simulink model "torqueBalancing2012b"  (Simulink 8.0)
settings: Solver=FixedStepDiscrete  StartTime=0.0  StopTime="CONFIG.SIMULATION_TIME "  FixedStep=CONFIG.Ts  RelTol=1e-3
InitFcn:
  | cd(fileparts(which(bdroot)));
  | initTorqueBalancing;
values from neighbouring files (symbols this model uses):
  baseToWorldRotationPort = ['/' WBT_modelName '/floatingBaseRotationMatrix:i']    [initTorqueBalancing.m]
  WBT_modelName = 'matlabTorqueBalancing'    [initTorqueBalancing.m]
undefined symbols (not defined in the file or in its folder): bVectorConstraints, CONFIG, ConstraintsMatrix, DiscIntNeverNeededParam, gain, references, reg, ROBOT_DOF, ROBOT_DOF_FOR_SIMULINK, sat, SM, sm, WBT_robotName
libraries: WBToolboxLibrary x114, simulink x11
(part 1 of 3)
settings Model: Creator=daniele  LastModifiedBy=DanielePucci
settings DebuggingCC: FcnCallInpInsideContextMsg=EnableAllAsWarning  FrameProcessingCompatibilityMsg=error
settings SFSimCC: SimParseCustomCode=off
settings CodeAppCC: CustomSymbolStrType=$N$R$M_T
settings GRTTargetCC: CodeReplacementLibrary=C89/C90 (ANSI)  CombineOutputUpdateFcns=off  GRTInterface=on

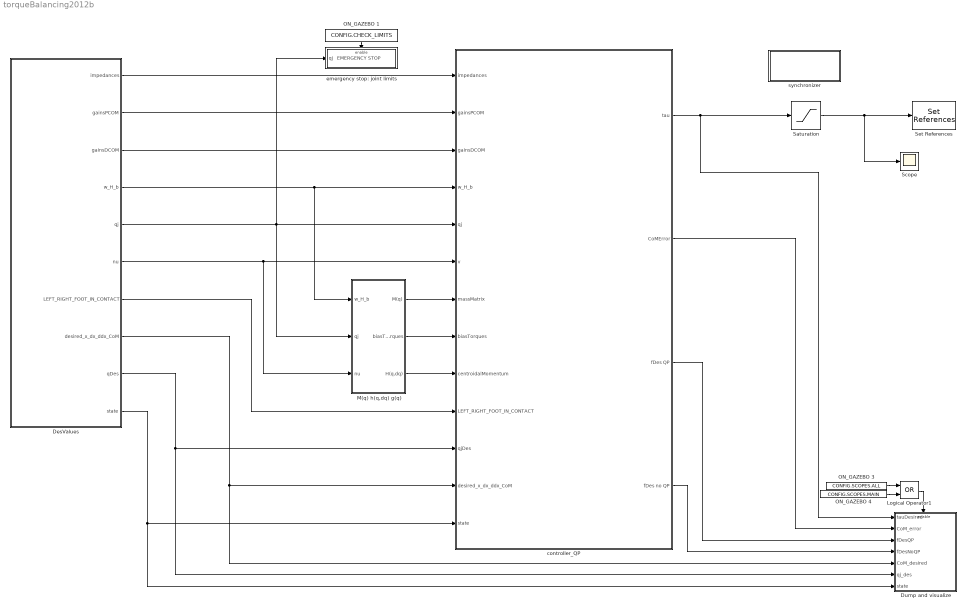
== system torqueBalancing2012b ==
  DesValues : Subsystem  Priority=-10
  Dump and visualize : Subsystem
  Logical Operator1 : Logic  Operator=OR  AllPortsSameDT=off  OutDataTypeStr=boolean
  M(q) h(q,dq) g(q) : Subsystem
  ON_GAZEBO 1 : Constant  Value=CONFIG.CHECK_LIMITS
  ON_GAZEBO 3 : Constant  Value=CONFIG.SCOPES.ALL
  ON_GAZEBO 4 : Constant  Value=CONFIG.SCOPES.MAIN
  Saturation : Saturate  UpperLimit=sat.torque  LowerLimit=-sat.torque
  Scope : Scope
      settings: TimeRange=auto  LimitDataPoints=on  MaxDataPoints=5000  SaveToWorkspace=off  YMin=-75.00000  YMax=75.00000  SampleTime=-1  DataFormat=Array
  Set References : WBToolboxLibrary/wholeBodyActuators/Set References  controlType=Torque  robotName=WBT_robotName  localName=WBT_modelName  wbiFile=WBT_wbiFilename  wbiList=WBT_wbiList
  controller_QP : Subsystem
  emergency stop: joint limits : Subsystem
  synchronizer : Subsystem
      mask Display: disp('SYNCHRONIZER')
  wires:
  M(q) h(q,dq) g(q)/1(M(q)) -> controller_QP/7(massMatrix)
  DesValues/5(qj) -> emergency stop: joint limits/1(qj   EMERGENCY STOP), controller_QP/5(qj), M(q) h(q,dq) g(q)/2(qj)
  M(q) h(q,dq) g(q)/2(biasTorques) -> controller_QP/8(biasTorques)
  M(q) h(q,dq) g(q)/3(H(q,dq)) -> controller_QP/9(centroidalMomentum)
  controller_QP/1("tau ") -> Dump and visualize/1(tauDesired), Saturation/1
  controller_QP/2(CoMError) -> Dump and visualize/2(CoM_error)
  DesValues/9(qDes) -> Dump and visualize/6(qj_des), controller_QP/11(qjDes)
  DesValues/7(LEFT_RIGHT_FOOT_IN_CONTACT) -> controller_QP/10(LEFT_RIGHT_FOOT_IN_CONTACT)
  DesValues/8(desired_x_dx_ddx_CoM) -> Dump and visualize/5(CoM_desired), controller_QP/12(desired_x_dx_ddx_CoM)
  DesValues/1(impedances) -> controller_QP/1(impedances)
  Saturation/1 -> Scope/1, Set References/1
  DesValues/4(w_H_b) -> M(q) h(q,dq) g(q)/1(w_H_b), controller_QP/4(w_H_b)
  DesValues/6(nu) -> controller_QP/6(v), M(q) h(q,dq) g(q)/3(nu)
  Logical Operator1/1 -> Dump and visualize/Enable
  DesValues/10(state) -> Dump and visualize/7(state), controller_QP/13("state ")
  controller_QP/4(fDes no QP) -> Dump and visualize/4(fDesNoQP)
  controller_QP/3(fDes QP) -> Dump and visualize/3(fDesQP)
  ON_GAZEBO 1/1 -> emergency stop: joint limits/Enable
  ON_GAZEBO 3/1 -> Logical Operator1/1
  ON_GAZEBO 4/1 -> Logical Operator1/2
  DesValues/2(gainsPCOM) -> controller_QP/2(gainsPCOM)
  DesValues/3(gainsDCOM) -> controller_QP/3(gainsDCOM)

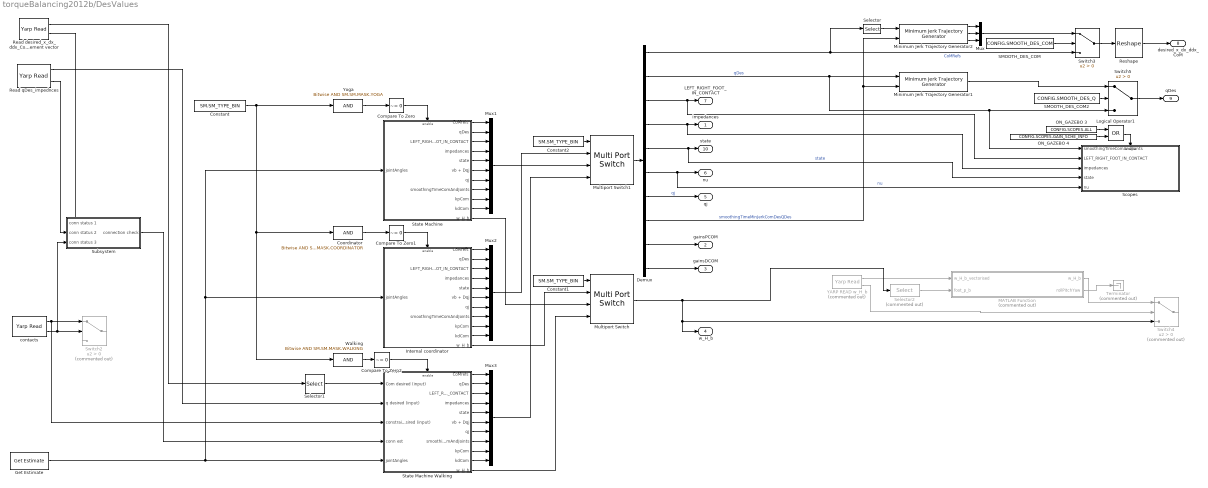
== system torqueBalancing2012b/DesValues ==
  Compare To Zero : simulink/Logic and Bit Operations/Compare To Zero  relop=~=  OutDataTypeStr=boolean
  Compare To Zero1 : simulink/Logic and Bit Operations/Compare To Zero  relop=~=  OutDataTypeStr=boolean
  Compare To Zero2 : simulink/Logic and Bit Operations/Compare To Zero  relop=~=  OutDataTypeStr=boolean
  Constant : Constant  Priority=-10  Value=SM.SM_TYPE_BIN  OutDataTypeStr=uint8
  Constant1 : Constant  Priority=-10  Value=SM.SM_TYPE_BIN  OutDataTypeStr=uint8
  Constant2 : Constant  Priority=-10  Value=SM.SM_TYPE_BIN  OutDataTypeStr=uint8
  Coordinator : simulink/Logic and Bit Operations/Bitwise Operator  logicop=AND  UseBitMask=on  BitMask=SM.SM.MASK.COORDINATOR  BitMaskRealWorld=Stored Integer
  Demux : Demux  Outputs=[9,ROBOT_DOF,2,ROBOT_DOF,1,ROBOT_DOF+6,ROBOT_DOF,1,3,3]
  Get Estimate : WBToolboxLibrary/wholeBodyStates/Get Estimate  estimateType=Joints Position  robotName=WBT_robotName  localName=WBT_modelName  wbiFile=WBT_wbiFilename  wbiList=WBT_wbiList
  Internal coordinator : Subsystem
  Logical Operator1 : Logic  Operator=OR  AllPortsSameDT=off  OutDataTypeStr=boolean
  MATLAB Function : MATLAB Function  Commented=on  TreatAsAtomicUnit=on
      settings: PermitHierarchicalResolution=ParametersOnly
  Minimum Jerk Trajectory Generator1 : WBToolboxLibrary/Utilities/Minimum Jerk Trajectory Generator  externalSettlingTime=on  settlingTime=1  sampleTime=CONFIG.Ts  firstDerivatives=off  secondDerivatives=off  explicitInitialValue=off
  Minimum Jerk Trajectory Generator2 : WBToolboxLibrary/Utilities/Minimum Jerk Trajectory Generator  externalSettlingTime=on  settlingTime=references.com.smoothingTime  sampleTime=CONFIG.Ts  firstDerivatives=on  secondDerivatives=on  explicitInitialValue=off
  Multiport Switch : MultiPortSwitch  DataPortOrder=Specify indices  DataPortIndices={1, 2, 4}
  Multiport Switch1 : MultiPortSwitch  DataPortOrder=Specify indices  DataPortIndices={1, 2, 4}
  Mux : Mux  Inputs=3
  Mux1 : Mux  Inputs=10
  Mux2 : Mux  Inputs=10
  Mux3 : Mux  Inputs=10
  ON_GAZEBO 3 : Constant  Value=CONFIG.SCOPES.ALL
  ON_GAZEBO 4 : Constant  Value=CONFIG.SCOPES.GAIN_SCHE_INFO
  Read desired_x_dx_ddx_CoM as 9 element vector : WBToolboxLibrary/Utilities/Yarp Read  portName=PORTS.COM_DES  signalSize=9  blocking=off  timestamp=off  autoconnect=off  errorOnConnection=on
  Read qDes_impednces : WBToolboxLibrary/Utilities/Yarp Read  portName=PORTS.Q_DES  signalSize=ROBOT_DOF  blocking=off  timestamp=off  autoconnect=off  errorOnConnection=on
  Reshape : Reshape  OutputDimensionality=Customize  OutputDimensions=[3,3]
  SMOOTH_DES_COM : Constant  Value=CONFIG.SMOOTH_DES_COM
  SMOOTH_DES_COM2 : Constant  Value=CONFIG.SMOOTH_DES_Q
  "Scopes  " : Subsystem
  Selector : Selector  InputPortWidth=9  IndexOptions=Index vector (dialog)  Indices=[1 2 3]  OutputSizes=1
  Selector1 : Selector  InputPortWidth=9  IndexOptions=Index vector (dialog)  Indices=[1 2 3]  OutputSizes=1
  Selector2 : Selector  Commented=on  NumberOfDimensions=2  InputPortWidth=3  IndexOptions=Index vector (dialog),Index vector (dialog)  Indices=[1 2 3],4  OutputSizes=1,1
  State Machine : Subsystem  Priority=-100
  State Machine Walking : Subsystem  Priority=-100
  Subsystem : Subsystem
  Switch2 : Switch  Commented=on  Criteria=u2 > Threshold
  Switch3 : Switch  Criteria=u2 > Threshold
  Switch4 : Switch  Commented=on  Criteria=u2 > Threshold
  Switch5 : Switch  Criteria=u2 > Threshold
  Terminator : Terminator  Commented=on
  Walking : simulink/Logic and Bit Operations/Bitwise Operator  logicop=AND  UseBitMask=on  BitMask=SM.SM.MASK.WALKING  BitMaskRealWorld=Stored Integer
  YARP READ w_H_b : WBToolboxLibrary/Utilities/Yarp Read  Commented=on  portName=[baseToWorldRotationPort]  signalSize=16  blocking=off  timestamp=off  autoconnect=off  errorOnConnection=on
  Yoga : simulink/Logic and Bit Operations/Bitwise Operator  logicop=AND  UseBitMask=on  BitMask=SM.SM.MASK.YOGA  BitMaskRealWorld=Stored Integer
  contacts : WBToolboxLibrary/Utilities/Yarp Read  portName=['/' WBT_modelName '/constraints:i']  signalSize=2  blocking=off  timestamp=off  autoconnect=off  errorOnConnection=on
  impedances : Outport
  gainsPCOM : Outport  Port=2
  gainsDCOM : Outport  Port=3
  w_H_b : Outport  Port=4
  qj : Outport  Port=5
  nu : Outport  Port=6
  LEFT_RIGHT_FOOT_IN_CONTACT : Outport  Port=7
  desired_x_dx_ddx_CoM : Outport  Port=8
  qDes : Outport  Port=9
  state : Outport  Port=10
  wires:
  Read desired_x_dx_ddx_CoM as 9 element vector/2 -> Subsystem/1(conn status 1)
  Read desired_x_dx_ddx_CoM as 9 element vector/1 -> Selector1/1
  Reshape/1 -> desired_x_dx_ddx_CoM/1
  Read qDes_impednces/2 -> Subsystem/2(conn status 2)
  contacts/2 -> Subsystem/3(conn status 3), Switch2/2
  Minimum Jerk Trajectory Generator2/1 -> Mux/1
  Minimum Jerk Trajectory Generator2/2 -> Mux/2
  Minimum Jerk Trajectory Generator2/3 -> Mux/3
  Switch3/1 -> Reshape/1
  SMOOTH_DES_COM/1 -> Switch3/2
  SMOOTH_DES_COM2/1 -> Switch5/2
  Switch5/1 -> qDes/1
  Constant/1 -> Walking/1, Coordinator/1, Yoga/1
  State Machine/3(LEFT_RIGHT_FOOT_IN_CONTACT) -> Mux1/3
  State Machine/2(qDes) -> Mux1/2
  State Machine/1(CoMrefs) -> Mux1/1
  Internal coordinator/1(CoMrefs) -> Mux2/1
  Internal coordinator/2(qDes) -> Mux2/2
  Internal coordinator/3(LEFT_RIGHT_FOOT_IN_CONTACT) -> Mux2/3
  State Machine/4(impedances) -> Mux1/4
  Internal coordinator/4(impedances) -> Mux2/4
  State Machine/5(state) -> Mux1/5
  Internal coordinator/5(state) -> Mux2/5
  Internal coordinator/6(vb + Dqj) -> Mux2/6
  Internal coordinator/7(qj) -> Mux2/7
  State Machine/6(vb + Dqj) -> Mux1/6
  State Machine/7(qj) -> Mux1/7
  Demux/7 -> qj/1  "qj"
  State Machine Walking/4(impedances) -> Mux3/4
  State Machine Walking/3(LEFT_RIGHT_FOOT_IN_CONTACT) -> Mux3/3
  State Machine Walking/5(state) -> Mux3/5
  State Machine Walking/6(vb + Dqj) -> Mux3/6
  State Machine Walking/1(CoMrefs) -> Mux3/1
  State Machine Walking/7(qj) -> Mux3/7
  Coordinator/1 -> Compare To Zero1/1
  Yoga/1 -> Compare To Zero/1
  Walking/1 -> Compare To Zero2/1
  Mux3/1 -> Multiport Switch1/4
  State Machine Walking/11(w_H_b) -> Multiport Switch/4
  Selector1/1 -> State Machine Walking/1(Com desired (input))
  Compare To Zero/1 -> State Machine/Enable
  Compare To Zero1/1 -> Internal coordinator/Enable
  Compare To Zero2/1 -> State Machine Walking/Enable
  Mux1/1 -> Multiport Switch1/3
  Mux2/1 -> Multiport Switch1/2
  State Machine/11(w_H_b) -> Multiport Switch/3
  Internal coordinator/11(w_H_b) -> Multiport Switch/2
  Read qDes_impednces/1 -> State Machine Walking/2(q desired (input))
  Subsystem/1(connection check) -> State Machine Walking/4(conn est)
  State Machine Walking/2(qDes) -> Mux3/2
  contacts/1 -> State Machine Walking/3(constraints desired (input)), Switch2/1
  YARP READ w_H_b/1 -> MATLAB Function/1(w_H_b_vectorised)
  MATLAB Function/1(w_H_b) -> Switch4/1
  Selector2/1 -> MATLAB Function/2(foot_p_b)
  Multiport Switch/1 -> Selector2/1, Switch4/3, w_H_b/1
  YARP READ w_H_b/2 -> Switch4/2
  MATLAB Function/2(rollPitchYaw) -> Terminator/1
  Demux/5 -> "Scopes  "/4(state), state/1  "state"
  Internal coordinator/8(smoothingTimeComAndJoints) -> Mux2/8
  State Machine Walking/8(smoothingTimeComAndJoints) -> Mux3/8
  State Machine/8(smoothingTimeComAndJoints) -> Mux1/8
  Demux/8 -> Minimum Jerk Trajectory Generator2/2, Minimum Jerk Trajectory Generator1/2  "smoothingTimeMinJerkComDesQDes"
  Logical Operator1/1 -> "Scopes  "/Enable
  Demux/1 -> Selector/1, Switch3/3  "CoMRefs"
  Mux/1 -> Switch3/1
  Selector/1 -> Minimum Jerk Trajectory Generator2/1
  Demux/2 -> Minimum Jerk Trajectory Generator1/1, "Scopes  "/1(smoothingTimeComAndJoints), Switch5/3  "qDes"
  Minimum Jerk Trajectory Generator1/1 -> Switch5/1
  ON_GAZEBO 3/1 -> Logical Operator1/1
  ON_GAZEBO 4/1 -> Logical Operator1/2
  Demux/6 -> nu/1, "Scopes  "/5(nu)  "nu"
  Get Estimate/1 -> State Machine/1(jointAngles), Internal coordinator/1(jointAngles), State Machine Walking/5(jointAngles)
  State Machine/9(kpCom) -> Mux1/9
  State Machine/10(kdCom) -> Mux1/10
  Internal coordinator/9(kpCom) -> Mux2/9
  Internal coordinator/10(kdCom) -> Mux2/10
  State Machine Walking/9(kpCom) -> Mux3/9
  State Machine Walking/10(kdCom) -> Mux3/10
  Multiport Switch1/1 -> Demux/1
  Demux/4 -> "Scopes  "/3(impedances), impedances/1
  Demux/3 -> "Scopes  "/2(LEFT_RIGHT_FOOT_IN_CONTACT), LEFT_RIGHT_FOOT_IN_CONTACT/1
  Demux/9 -> gainsPCOM/1
  Demux/10 -> gainsDCOM/1
  Constant1/1 -> Multiport Switch/1
  Constant2/1 -> Multiport Switch1/1

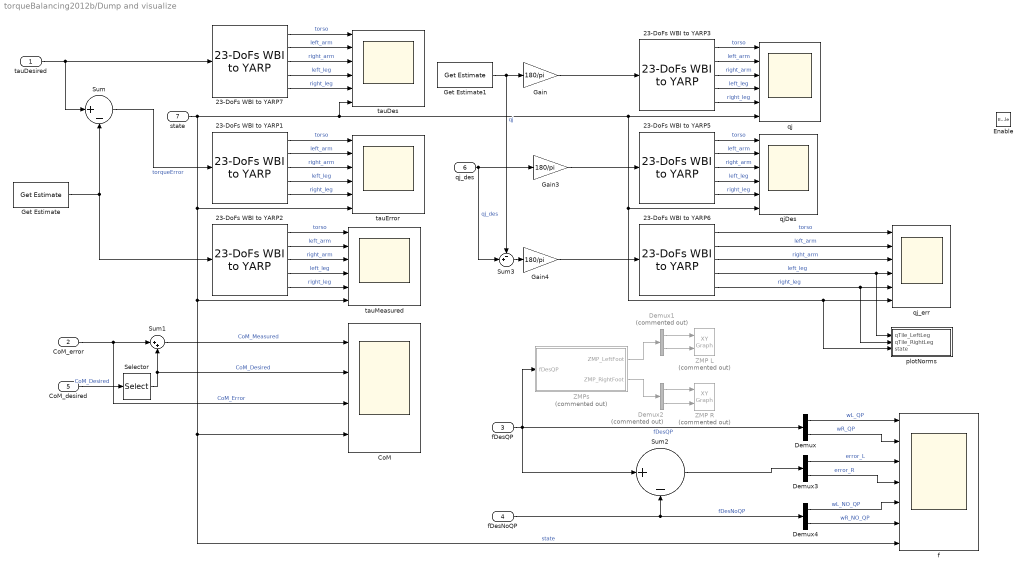
== system torqueBalancing2012b/Dump and visualize ==
  tauDesired : Inport
  CoM_error : Inport  Port=2
  fDesQP : Inport  Port=3
  fDesNoQP : Inport  Port=4
  CoM_desired : Inport  Port=5
  qj_des : Inport  Port=6
  state : Inport  Port=7
  Enable : EnablePort
  23-DoFs WBI to YARP{1..3,5..7} (6 alike) : WBToolboxLibrary/Utilities/23-DoFs WBI to YARP
  CoM : Scope  NumInputPorts=4
      settings: TimeRange=400  ShowLegends=on  MaxDataPoints=5000  SaveToWorkspace=off  SaveName=CoM_data  YMin=-0.89345~-0.34739~-1.03525~0.625  YMax=1.44665~1.31967~1.03732~4.375  SampleTime=-1
  Demux : Demux  Outputs=2
  Demux1 : Demux  Commented=on  Outputs=2
  Demux2 : Demux  Commented=on  Outputs=2
  Demux3 : Demux  Outputs=2
  Demux4 : Demux  Outputs=2
  Gain : Gain  Gain=180/pi
  Gain3 : Gain  Gain=180/pi
  Gain4 : Gain  Gain=180/pi
  Get Estimate : WBToolboxLibrary/wholeBodyStates/Get Estimate  estimateType=Joints Torque  robotName=WBT_robotName  localName=WBT_modelName  wbiFile=WBT_wbiFilename  wbiList=WBT_wbiList
  Get Estimate1 : WBToolboxLibrary/wholeBodyStates/Get Estimate  estimateType=Joints Position  robotName=WBT_robotName  localName=WBT_modelName  wbiFile=WBT_wbiFilename  wbiList=WBT_wbiList
  Selector : Selector  NumberOfDimensions=2  IndexOptions=Index vector (dialog),Index vector (dialog)  Indices=[1:3],1  OutputSizes=1,1
  Sum : Sum  Inputs=|+-
  Sum1 : Sum  Inputs=|++
  Sum2 : Sum  Inputs=|+-
  Sum3 : Sum  Inputs=-+|
  ZMP L : simulink/Sinks/XY Graph  Commented=on  xmin=gain.footSize(1,1)  xmax=gain.footSize(1,2)  ymin=gain.footSize(2,1)  ymax=gain.footSize(2,2)  st=-1
  ZMP R : simulink/Sinks/XY Graph  Commented=on  xmin=gain.footSize(1,1)  xmax=gain.footSize(1,2)  ymin=gain.footSize(2,1)  ymax=gain.footSize(2,2)  st=-1
  ZMPs : Subsystem  Commented=on
  f : Scope  NumInputPorts=7
      settings: TimeRange=40  MaxDataPoints=5000  SaveToWorkspace=off  SaveName=ScopeData2  YMin=-58.62138~-58.62138~-58.62138~-58.62138~-58.62138~-58.62138~-58.62138  YMax=275.46472~275.46472~275.46472~275.46472~275.46472~275.46472~275.46472  SampleTime=-1  DataFormat=Array
  plotNorms : Subsystem
  qj : Scope  NumInputPorts=6
      settings: TimeRange=40  ShowLegends=on  MaxDataPoints=5000  SaveToWorkspace=off  SaveName=qj_and_v  YMin=-27.84492~-27.84492~-27.84492~-27.84492~-27.84492~-27.84492  YMax=29.50386~29.50386~29.50386~29.50386~29.50386~29.50386  SampleTime=-1
  qjDes : Scope  NumInputPorts=6
      settings: TimeRange=40  ShowLegends=on  MaxDataPoints=5000  SaveToWorkspace=off  SaveName=qj_and_v3  YMin=-30.77436~-30.77436~-30.77436~-30.77436~-30.77436~-30.77436  YMax=32.14439~32.14439~32.14439~32.14439~32.14439~32.14439  SampleTime=-1
  qj_err : Scope  NumInputPorts=6
      settings: TimeRange=40  ShowLegends=on  MaxDataPoints=5000  SaveToWorkspace=off  SaveName=qj_and_v4  YMin=-19.07921~-19.07921~-19.07921~-19.07921~-19.07921~-19.07921  YMax=25.04716~25.04716~25.04716~25.04716~25.04716~25.04716  SampleTime=-1
  tauDes : Scope  NumInputPorts=6
      settings: TimeRange=14  ShowLegends=on  MaxDataPoints=5000  SaveToWorkspace=off  SaveName=tauDes  YMin=-11.78546~-11.78546~-11.78546~-11.78546~-11.78546~-11.78546  YMax=8.52242~8.52242~8.52242~8.52242~8.52242~8.52242  SampleTime=-1
  tauError : Scope  NumInputPorts=6
      settings: TimeRange=90  ShowLegends=on  MaxDataPoints=5000  SaveToWorkspace=off  SaveName=tauError  YMin=-9.6915~-5.81436~-6.54838~-48.80934~-49.21526~-0.5  YMax=9.49753~5.53968~7.62852~37.43254~39.21906~14.5  SampleTime=-1
  tauMeasured : Scope  NumInputPorts=6
      settings: TimeRange=14  ShowLegends=on  MaxDataPoints=5000  SaveToWorkspace=off  SaveName=tauMeasured  YMin=-10.14812~-10.14812~-10.14812~-10.14812~-10.14812~-10.14812  YMax=9.97513~9.97513~9.97513~9.97513~9.97513~9.97513  SampleTime=-1
  wires:
  CoM_error/1 -> Sum1/1, CoM/3  "CoM_Error"
  CoM_desired/1 -> Selector/1  "CoM_Desired"
  Sum1/1 -> CoM/1  "CoM_Measured"
  Get Estimate1/1 -> Sum3/1, Gain/1  "qj"
  Gain/1 -> 23-DoFs WBI to YARP3/1
  23-DoFs WBI to YARP3/5 -> qj/5  "right_leg"
  23-DoFs WBI to YARP3/1 -> qj/1  "torso"
  23-DoFs WBI to YARP3/2 -> qj/2  "left_arm"
  23-DoFs WBI to YARP3/4 -> qj/4  "left_leg"
  23-DoFs WBI to YARP3/3 -> qj/3  "right_arm"
  fDesQP/1 -> Demux/1, ZMPs/1(fDesQP), Sum2/1  "fDesQP"
  ZMPs/1(ZMP_LeftFoot) -> Demux1/1
  ZMPs/2(ZMP_RightFoot) -> Demux2/1
  Demux1/1 -> ZMP L/1
  Demux1/2 -> ZMP L/2
  Demux2/1 -> ZMP R/1
  Demux2/2 -> ZMP R/2
  Sum2/1 -> Demux3/1
  fDesNoQP/1 -> Demux4/1, Sum2/2  "fDesNoQP"
  tauDesired/1 -> 23-DoFs WBI to YARP7/1, Sum/1
  Get Estimate/1 -> 23-DoFs WBI to YARP2/1, Sum/2
  23-DoFs WBI to YARP7/5 -> tauDes/5  "right_leg"
  23-DoFs WBI to YARP7/1 -> tauDes/1  "torso"
  23-DoFs WBI to YARP7/2 -> tauDes/2  "left_arm"
  23-DoFs WBI to YARP7/4 -> tauDes/4  "left_leg"
  23-DoFs WBI to YARP7/3 -> tauDes/3  "right_arm"
  23-DoFs WBI to YARP1/5 -> tauError/5  "right_leg"
  23-DoFs WBI to YARP1/1 -> tauError/1  "torso"
  23-DoFs WBI to YARP1/2 -> tauError/2  "left_arm"
  23-DoFs WBI to YARP1/4 -> tauError/4  "left_leg"
  23-DoFs WBI to YARP1/3 -> tauError/3  "right_arm"
  Sum/1 -> 23-DoFs WBI to YARP1/1  "torqueError"
  23-DoFs WBI to YARP2/5 -> tauMeasured/5  "right_leg"
  23-DoFs WBI to YARP2/1 -> tauMeasured/1  "torso"
  23-DoFs WBI to YARP2/2 -> tauMeasured/2  "left_arm"
  23-DoFs WBI to YARP2/4 -> tauMeasured/4  "left_leg"
  23-DoFs WBI to YARP2/3 -> tauMeasured/3  "right_arm"
  qj_des/1 -> Sum3/2, Gain3/1  "qj_des"
  Gain3/1 -> 23-DoFs WBI to YARP5/1
  23-DoFs WBI to YARP5/5 -> qjDes/5  "right_leg"
  23-DoFs WBI to YARP5/1 -> qjDes/1  "torso"
  23-DoFs WBI to YARP5/2 -> qjDes/2  "left_arm"
  23-DoFs WBI to YARP5/4 -> qjDes/4  "left_leg"
  23-DoFs WBI to YARP5/3 -> qjDes/3  "right_arm"
  Gain4/1 -> 23-DoFs WBI to YARP6/1
  23-DoFs WBI to YARP6/5 -> plotNorms/2(qTile_RightLeg), qj_err/5  "right_leg"
  23-DoFs WBI to YARP6/1 -> qj_err/1  "torso"
  23-DoFs WBI to YARP6/2 -> qj_err/2  "left_arm"
  23-DoFs WBI to YARP6/4 -> plotNorms/1(qTile_LeftLeg), qj_err/4  "left_leg"
  23-DoFs WBI to YARP6/3 -> qj_err/3  "right_arm"
  Sum3/1 -> Gain4/1
  Selector/1 -> Sum1/2, CoM/2  "CoM_Desired"
  state/1 -> tauDes/6, plotNorms/3(state), qj_err/6, qjDes/6, qj/6, f/7, CoM/4, tauMeasured/6, tauError/6  "state"
  Demux/1 -> f/1  "wL_QP"
  Demux/2 -> f/2  "wR_QP"
  Demux3/1 -> f/3  "error_L"
  Demux3/2 -> f/4  "error_R"
  Demux4/1 -> f/5  "wL_NO_QP"
  Demux4/2 -> f/6  "wR_NO_QP"

== system torqueBalancing2012b/M(q) h(q,dq) g(q) ==
  w_H_b : Inport
  qj : Inport  Port=2
  nu : Inport  Port=3
  Centroidal Momentum : WBToolboxLibrary/wholeBodyModel/Dynamics/Centroidal Momentum  robotName=WBT_robotName  localName=WBT_modelName  wbiFile=WBT_wbiFilename  wbiList=WBT_wbiList
  "CoM6D ->  CoMXYZ1" : Selector  InputPortWidth=6+ROBOT_DOF  IndexOptions=Index vector (dialog)  Indices=[7:6+ROBOT_DOF]  OutputSizes=1
  "CoM6D ->  CoMXYZ2" : Selector  InputPortWidth=6+ROBOT_DOF  IndexOptions=Index vector (dialog)  Indices=[1 2 3 4 5 6]  OutputSizes=1
  Get Bias Forces : WBToolboxLibrary/wholeBodyModel/Dynamics/Get Bias Forces  robotName=WBT_robotName  localName=WBT_modelName  wbiFile=WBT_wbiFilename  wbiList=WBT_wbiList  explicitGravity=off
  Mass Matrix : WBToolboxLibrary/wholeBodyModel/Dynamics/Mass Matrix  robotName=WBT_robotName  localName=WBT_modelName  wbiFile=WBT_wbiFilename  wbiList=WBT_wbiList
  M(q) : Outport
  biasTorques : Outport  Port=2
  H(q,dq) : Outport  Port=3
  wires:
  Mass Matrix/1 -> M(q)/1
  Centroidal Momentum/1 -> H(q,dq)/1
  Get Bias Forces/1 -> biasTorques/1
  w_H_b/1 -> Centroidal Momentum/1, Get Bias Forces/1, Mass Matrix/1
  qj/1 -> Centroidal Momentum/2, Get Bias Forces/2, Mass Matrix/2
  "CoM6D ->  CoMXYZ2"/1 -> Centroidal Momentum/3, Get Bias Forces/3
  "CoM6D ->  CoMXYZ1"/1 -> Get Bias Forces/4, Centroidal Momentum/4
  nu/1 -> "CoM6D ->  CoMXYZ1"/1, "CoM6D ->  CoMXYZ2"/1

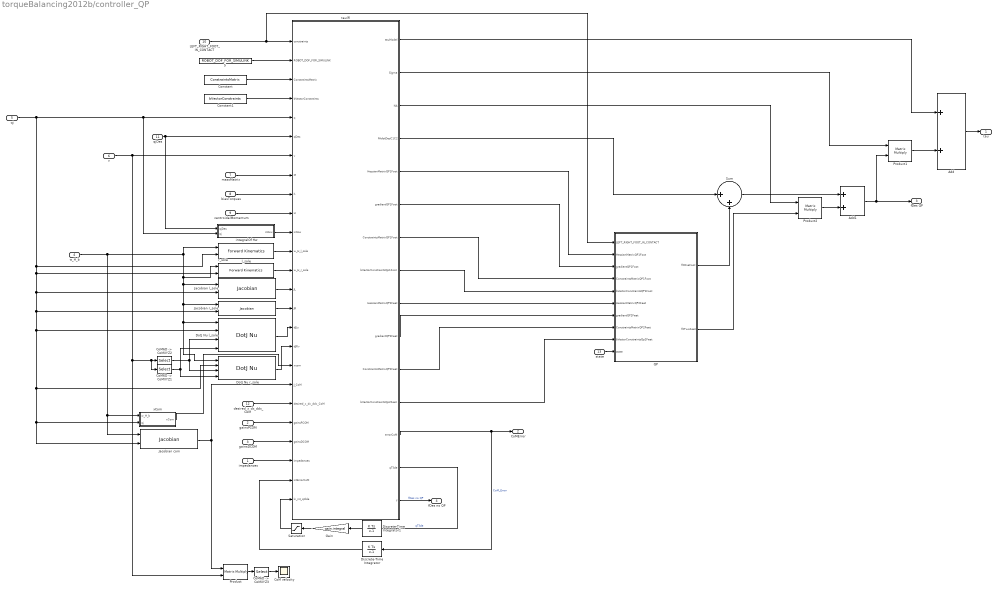
== system torqueBalancing2012b/controller_QP ==
  impedances : Inport
  gainsPCOM : Inport  Port=2
  gainsDCOM : Inport  Port=3
  w_H_b : Inport  Port=4
  qj : Inport  Port=5
  v : Inport  Port=6
  massMatrix : Inport  Port=7
  biasTorques : Inport  Port=8
  centroidalMomentum : Inport  Port=9
  LEFT_RIGHT_FOOT_IN_CONTACT : Inport  Port=10
  qjDes : Inport  Port=11
  desired_x_dx_ddx_CoM : Inport  Port=12
  "state " : Inport  Port=13
  "    5" : Constant  Value=ROBOT_DOF_FOR_SIMULINK
  Add : Sum
  Add1 : Sum
  CoM velocity : Scope
      settings: TimeRange=auto  MaxDataPoints=5000  SaveToWorkspace=off  SaveName=ScopeData3  YMin=-0.13469  YMax=0.38733  SampleTime=-1
  "CoM6D ->  CoMXYZ1" : Selector  InputPortWidth=6+ROBOT_DOF  IndexOptions=Index vector (dialog)  Indices=[7:6+ROBOT_DOF]  OutputSizes=1
  "CoM6D ->  CoMXYZ2" : Selector  InputPortWidth=6+ROBOT_DOF  IndexOptions=Index vector (dialog)  Indices=[1 2 3 4 5 6]  OutputSizes=1
  "CoM6D ->  CoMXYZ3" : Selector  InputPortWidth=6  IndexOptions=Index vector (dialog)  Indices=[1 2 3]  OutputSizes=1
  Constant : Constant  Value=ConstraintsMatrix
  Constant1 : Constant  Value=bVectorConstraints
  Discrete-Time Integrator : DiscreteIntegrator  InitialCondition=[0 0 0]  SampleTime=CONFIG.Ts  ICPrevOutput=DiscIntNeverNeededParam  ICPrevScaledInput=DiscIntNeverNeededParam
  Discrete-Time Integrator1 : DiscreteIntegrator  InitialCondition=zeros(ROBOT_DOF,1)  SampleTime=CONFIG.Ts  ICPrevOutput=DiscIntNeverNeededParam  ICPrevScaledInput=DiscIntNeverNeededParam
  "DotJ Nu l_sole " : WBToolboxLibrary/wholeBodyModel/Jacobians/DotJ Nu  frameName='l_sole'  robotName=WBT_robotName  localName=WBT_modelName  wbiFile=WBT_wbiFilename  wbiList=WBT_wbiList
  "DotJ Nu r_sole " : WBToolboxLibrary/wholeBodyModel/Jacobians/DotJ Nu  frameName='r_sole'  robotName=WBT_robotName  localName=WBT_modelName  wbiFile=WBT_wbiFilename  wbiList=WBT_wbiList
  Gain : Gain  Gain=gain.integral
  Jacobian com : WBToolboxLibrary/wholeBodyModel/Jacobians/Jacobian  frameName='com'  robotName=WBT_robotName  localName=WBT_modelName  wbiFile=WBT_wbiFilename  wbiList=WBT_wbiList
  Jacobian l_sole : WBToolboxLibrary/wholeBodyModel/Jacobians/Jacobian  frameName='l_sole'  robotName=WBT_robotName  localName=WBT_modelName  wbiFile=WBT_wbiFilename  wbiList=WBT_wbiList
  Jacobian r_sole : WBToolboxLibrary/wholeBodyModel/Jacobians/Jacobian  frameName='r_sole'  robotName=WBT_robotName  localName=WBT_modelName  wbiFile=WBT_wbiFilename  wbiList=WBT_wbiList
  Product : Product  Multiplication=Matrix(*)
  Product1 : Product  Multiplication=Matrix(*)
  Product2 : Product  Multiplication=Matrix(*)
  QP : Subsystem
  Saturation : Saturate  UpperLimit=sat.integral  LowerLimit=-sat.integral
  Sum : Sum  Inputs=|++
  integralOf Hw : Subsystem
  l_sole : WBToolboxLibrary/wholeBodyModel/Kinematics/Forward Kinematics  frameName='l_sole'  robotName=WBT_robotName  localName=WBT_modelName  wbiFile=WBT_wbiFilename  wbiList=WBT_wbiList
  r_sole : WBToolboxLibrary/wholeBodyModel/Kinematics/Forward Kinematics  frameName='r_sole'  robotName=WBT_robotName  localName=WBT_modelName  wbiFile=WBT_wbiFilename  wbiList=WBT_wbiList
  "tau(f) " : MATLAB Function  TreatAsAtomicUnit=on
      settings: PermitHierarchicalResolution=ParametersOnly
  xCom : Subsystem
  "tau " : Outport
  CoMError : Outport  Port=2
  fDes QP : Outport  Port=3
  fDes no QP : Outport  Port=4
  wires:
  LEFT_RIGHT_FOOT_IN_CONTACT/1 -> QP/1(LEFT_RIGHT_FOOT_IN_CONTACT), "tau(f) "/1(constraints)
  Discrete-Time Integrator/1 -> "tau(f) "/24(intErrorCoM)
  "tau(f) "/13(errorCoM) -> CoMError/1, Discrete-Time Integrator/1  "CoM_Error"
  Discrete-Time Integrator1/1 -> Gain/1
  "tau(f) "/14(qTilde) -> Discrete-Time Integrator1/1  "qTilde"
  Gain/1 -> Saturation/1
  Saturation/1 -> "tau(f) "/25(ki_int_qtilde)
  qj/1 -> l_sole/2, xCom/2(qj), Jacobian com/2, "DotJ Nu r_sole "/2, "DotJ Nu l_sole "/2, Jacobian r_sole/2, Jacobian l_sole/2, r_sole/2, integralOf Hw/2(qj), "tau(f) "/5(q)
  qjDes/1 -> integralOf Hw/1(qjDes), "tau(f) "/6(qDes)
  massMatrix/1 -> "tau(f) "/8(M)
  biasTorques/1 -> "tau(f) "/9(h)
  desired_x_dx_ddx_CoM/1 -> "tau(f) "/20(desired_x_dx_ddx_CoM)
  impedances/1 -> "tau(f) "/23(impedances)
  centroidalMomentum/1 -> "tau(f) "/10(H)
  r_sole/1 -> "tau(f) "/13(w_H_r_sole)
  l_sole/1 -> "tau(f) "/12(w_H_l_sole)
  Jacobian l_sole/1 -> "tau(f) "/14(JL)
  Jacobian r_sole/1 -> "tau(f) "/15(JR)
  Jacobian com/1 -> Product/1, "tau(f) "/19(J_CoM)
  "tau(f) "/5(HessianMatrixQP1Foot) -> QP/2(HessianMatrixQP1Foot)
  "tau(f) "/6(gradientQP1Foot) -> QP/3(gradientQP1Foot)
  "tau(f) "/9(HessianMatrixQP2Feet) -> QP/6(HessianMatrixQP2Feet)
  "tau(f) "/10(gradientQP2Feet) -> QP/7(gradientQP2Feet)
  "tau(f) "/11(ConstraintsMatrixQP2Feet) -> QP/8(ConstraintsMatrixQP2Feet)
  "tau(f) "/12(bVectorConstraintsQp2Feet) -> QP/9(bVectorConstraintsQp2Feet)
  "tau(f) "/4(fHdotDesC1C2) -> Sum/1
  QP/1(f0OneFoot) -> Sum/2
  Product1/1 -> Add/2
  "tau(f) "/1(tauModel) -> Add/1
  Add/1 -> "tau "/1
  Add1/1 -> fDes QP/1, Product1/2
  "    5"/1 -> "tau(f) "/2(ROBOT_DOF_FOR_SIMULINK)
  Constant/1 -> "tau(f) "/3(ConstraintsMatrix)
  Constant1/1 -> "tau(f) "/4(bVectorConstraints)
  "tau(f) "/7(ConstraintsMatrixQP1Foot) -> QP/4(ConstraintsMatrixQP1Foot)
  "tau(f) "/8(bVectorConstraintsQp1Foot) -> QP/5(bVectorConstraintsQP1Foot)
  Sum/1 -> Add1/1
  Product2/1 -> Add1/2
  "tau(f) "/3(NA) -> Product2/1
  "tau(f) "/2(Sigma) -> Product1/1
  "tau(f) "/15(f) -> fDes no QP/1  "fDes no QP"
  "DotJ Nu l_sole "/1 -> "tau(f) "/16(dJLv)
  "DotJ Nu r_sole "/1 -> "tau(f) "/17(dJRv)
  xCom/1(xCom) -> "tau(f) "/18(xcom)
  "CoM6D ->  CoMXYZ2"/1 -> "DotJ Nu r_sole "/3, "DotJ Nu l_sole "/3
  "CoM6D ->  CoMXYZ1"/1 -> "DotJ Nu r_sole "/4, "DotJ Nu l_sole "/4
  w_H_b/1 -> xCom/1(w_H_b), Jacobian com/1, r_sole/1, "DotJ Nu r_sole "/1, "DotJ Nu l_sole "/1, Jacobian r_sole/1, Jacobian l_sole/1, l_sole/1
  QP/2(f0TwoFeet) -> Product2/2
  integralOf Hw/1(intHw) -> "tau(f) "/11(intHw)
  "state "/1 -> QP/10(state)
  v/1 -> Product/2, "CoM6D ->  CoMXYZ1"/1, "CoM6D ->  CoMXYZ2"/1, "tau(f) "/7(v)
  Product/1 -> "CoM6D ->  CoMXYZ3"/1
  "CoM6D ->  CoMXYZ3"/1 -> CoM velocity/1
  gainsPCOM/1 -> "tau(f) "/21(gainsPCOM)
  gainsDCOM/1 -> "tau(f) "/22(gainsDCOM)

== system torqueBalancing2012b/emergency stop: joint limits ==
  qj   EMERGENCY STOP : Inport
  Enable : EnablePort
  Assertion : Assertion
  Get Limits : WBToolboxLibrary/wholeBodyStates/Get Limits  limitsType=Position  robotName=WBT_robotName  localName=WBT_modelName  wbiFile=WBT_wbiFilename  wbiList=WBT_wbiList
  MATLAB Function : MATLAB Function  TreatAsAtomicUnit=on
      settings: PermitHierarchicalResolution=ParametersOnly
  index1 : Constant  Value=0.01  VectorParams1D=off
  wires:
  Get Limits/1 -> MATLAB Function/1(umin)
  Get Limits/2 -> MATLAB Function/2(umax)
  index1/1 -> MATLAB Function/4(tol)
  qj   EMERGENCY STOP/1 -> MATLAB Function/3(u)
  MATLAB Function/1(inRange) -> Assertion/1

== system torqueBalancing2012b/synchronizer ==
  GAZEBO_SYNCHRONIZER : Subsystem
  Logical Operator : Logic  Operator=NOT  AllPortsSameDT=off  OutDataTypeStr=boolean
  "ON_GAZEBO " : Constant  Value=CONFIG.ON_GAZEBO
  REAL_TIME_SYNC : Subsystem
  wires:
  Logical Operator/1 -> REAL_TIME_SYNC/Enable
  "ON_GAZEBO "/1 -> GAZEBO_SYNCHRONIZER/Enable, Logical Operator/1

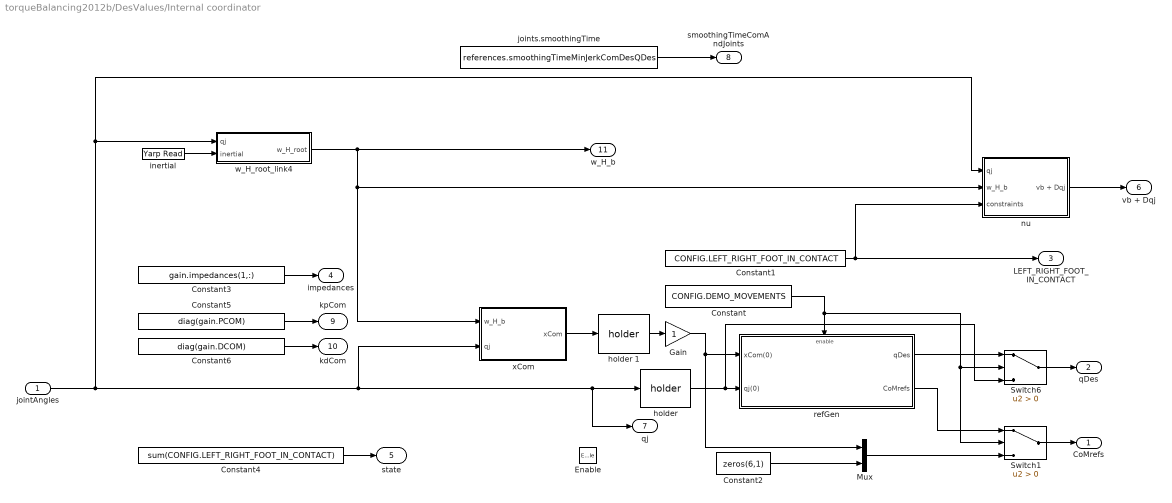
== system torqueBalancing2012b/DesValues/Internal coordinator ==
  jointAngles : Inport
  Enable : EnablePort
  Constant : Constant  Value=CONFIG.DEMO_MOVEMENTS
  Constant1 : Constant  Value=CONFIG.LEFT_RIGHT_FOOT_IN_CONTACT
  Constant2 : Constant  Value=zeros(6,1)
  Constant3 : Constant  Value=gain.impedances(1,:)
  Constant4 : Constant  Value=sum(CONFIG.LEFT_RIGHT_FOOT_IN_CONTACT)
  Constant5 : Constant  Value=diag(gain.PCOM)
  Constant6 : Constant  Value=diag(gain.DCOM)
  Gain : Gain
  Mux : Mux  Inputs=2
  Switch1 : Switch  Criteria=u2 > Threshold
  Switch6 : Switch  Criteria=u2 > Threshold
  "holder " : WBToolboxLibrary/Utilities/holder 
  holder 1 : WBToolboxLibrary/Utilities/holder 
  inertial : WBToolboxLibrary/Utilities/Yarp Read  portName=PORTS.IMU  signalSize=12  blocking=off  timestamp=off  autoconnect=on  errorOnConnection=on
  joints.smoothingTime : Constant  Value=references.smoothingTimeMinJerkComDesQDes
  nu : Subsystem
  refGen : Subsystem
  w_H_root_link4 : Subsystem  mask{link_name='l_sole'}
      mask prompts: link_name "link name"
      mask help:
      | This block evaluates the homogeneous transformation between the world and the root link, i.e. ^wH_b. It assumes that the link specified by the variable 'link_name' has a constant position
      | w.r.t. an inertial frame, but it can rotate arbitrarily. This rotation is retrived from the IMU sensor.
      mask Display:
      | str = strrep(link_name, '_','\_');
      | port_label('output',1,['{}^{',str '}H_{root}'],'texmode','on')
      | clear str;
      | 
      | port_label('input',1,'q_j','texmode','on')
      | 
      | port_label('input',2,'inertial','texmode','on')
  xCom : Subsystem
  CoMrefs : Outport
  qDes : Outport  Port=2
  LEFT_RIGHT_FOOT_IN_CONTACT : Outport  Port=3
  impedances : Outport  Port=4
  state : Outport  Port=5
  vb + Dqj : Outport  Port=6
  qj : Outport  Port=7
  smoothingTimeComAndJoints : Outport  Port=8
  kpCom : Outport  Port=9
  kdCom : Outport  Port=10
  w_H_b : Outport  Port=11
  wires:
  Constant1/1 -> nu/3("constraints "), LEFT_RIGHT_FOOT_IN_CONTACT/1
  "holder "/1 -> Switch6/3, refGen/2(qj(0))
  Constant/1 -> Switch1/2, Switch6/2, refGen/Enable
  Switch6/1 -> qDes/1
  Switch1/1 -> CoMrefs/1
  refGen/1(qDes) -> Switch6/1
  refGen/2(CoMrefs) -> Switch1/1
  Mux/1 -> Switch1/3
  Constant2/1 -> Mux/2
  Constant3/1 -> impedances/1
  Constant4/1 -> state/1
  nu/1(vb + Dqj) -> vb + Dqj/1
  holder 1/1 -> Gain/1
  w_H_root_link4/1(w_H_root) -> nu/2(w_H_b), xCom/1(w_H_b), w_H_b/1
  xCom/1(xCom) -> holder 1/1
  joints.smoothingTime/1 -> smoothingTimeComAndJoints/1
  jointAngles/1 -> w_H_root_link4/1(qj), nu/1(qj), xCom/2(qj), "holder "/1, qj/1
  inertial/1 -> w_H_root_link4/2(inertial)
  Constant5/1 -> kpCom/1
  Constant6/1 -> kdCom/1
  Gain/1 -> Mux/1, refGen/1(xCom(0))

== system torqueBalancing2012b/DesValues/Scopes   ==
  smoothingTimeComAndJoints : Inport
  LEFT_RIGHT_FOOT_IN_CONTACT : Inport  Port=2
  impedances : Inport  Port=3
  state : Inport  Port=4
  nu : Inport  Port=5
  Enable : EnablePort
  23-DoFs WBI to YARP1 : WBToolboxLibrary/Utilities/23-DoFs WBI to YARP
  23-DoFs WBI to YARP5 : WBToolboxLibrary/Utilities/23-DoFs WBI to YARP
  Demux : Demux  Outputs=2
  Gain : Gain  Gain=180/pi
  Gain1 : Gain  Gain=180/pi
  Impedances(t) : Scope  NumInputPorts=6
      settings: TimeRange=auto  ShowLegends=on  MaxDataPoints=5000  SaveToWorkspace=off  SaveName=ScopeData3  YMin=27.5~27.5~27.5~27.5~27.5~27.5  YMax=52.5~52.5~52.5~52.5~52.5~52.5  SampleTime=-1
  Left right foot in contact : Scope
      settings: TimeRange=auto  ShowLegends=on  MaxDataPoints=5000  SaveToWorkspace=off  YMin=-0.09603  YMax=1.127  SampleTime=-1
  Selector1 : Selector  InputPortWidth=6+ROBOT_DOF  IndexOptions=Index vector (dialog)  Indices=[7:6+ROBOT_DOF]  OutputSizes=1
  Selector2 : Selector  InputPortWidth=6+ROBOT_DOF  IndexOptions=Index vector (dialog)  Indices=[1:6]  OutputSizes=1
  jointsSmoothingTime : Scope  NumInputPorts=2
      settings: TimeRange=auto  MaxDataPoints=5000  SaveToWorkspace=off  SaveName=ScopeData4  YMin=-0.375~-0.375  YMax=13.375~13.375  SampleTime=-1
  linear and angular  base velocity : Scope  NumInputPorts=3
      settings: TimeRange=auto  ShowLegends=on  MaxDataPoints=5000  SaveToWorkspace=off  SaveName=ScopeData2  YMin=-0.04416~-19.05827~-0.5  YMax=0.05054~20.49714~14.5  SampleTime=-1
  "qjDot(t) " : Scope  NumInputPorts=6
      settings: TimeRange=60  ShowLegends=on  MaxDataPoints=5000  SaveToWorkspace=off  YMin=-20.50153~-13.93091~-14.07118~-86.04652~-89.15901~-0.5  YMax=20.29706~17.04678~16.66387~63.96852~62.87068~14.5  SampleTime=-1
  wires:
  state/1 -> "qjDot(t) "/6, linear and angular  base velocity/3, Impedances(t)/6, jointsSmoothingTime/2  "state"
  LEFT_RIGHT_FOOT_IN_CONTACT/1 -> Left right foot in contact/1  "Left right foot in contact"
  impedances/1 -> 23-DoFs WBI to YARP5/1
  smoothingTimeComAndJoints/1 -> jointsSmoothingTime/1  "smoothingTimeComAndJoints"
  23-DoFs WBI to YARP5/4 -> Impedances(t)/4  "left_leg"
  23-DoFs WBI to YARP5/5 -> Impedances(t)/5  "right_leg"
  23-DoFs WBI to YARP5/3 -> Impedances(t)/3  "right_arm"
  23-DoFs WBI to YARP5/1 -> Impedances(t)/1  "torso"
  23-DoFs WBI to YARP5/2 -> Impedances(t)/2  "left_arm"
  Selector1/1 -> Gain/1
  23-DoFs WBI to YARP1/4 -> "qjDot(t) "/4  "left_leg"
  23-DoFs WBI to YARP1/5 -> "qjDot(t) "/5  "right_leg"
  23-DoFs WBI to YARP1/3 -> "qjDot(t) "/3  "right_arm"
  23-DoFs WBI to YARP1/1 -> "qjDot(t) "/1  "torso"
  23-DoFs WBI to YARP1/2 -> "qjDot(t) "/2  "left_arm"
  nu/1 -> Selector1/1, Selector2/1
  Selector2/1 -> Demux/1
  Demux/1 -> linear and angular  base velocity/1  "vb"
  Demux/2 -> Gain1/1  "wb"
  Gain/1 -> 23-DoFs WBI to YARP1/1
  Gain1/1 -> linear and angular  base velocity/2

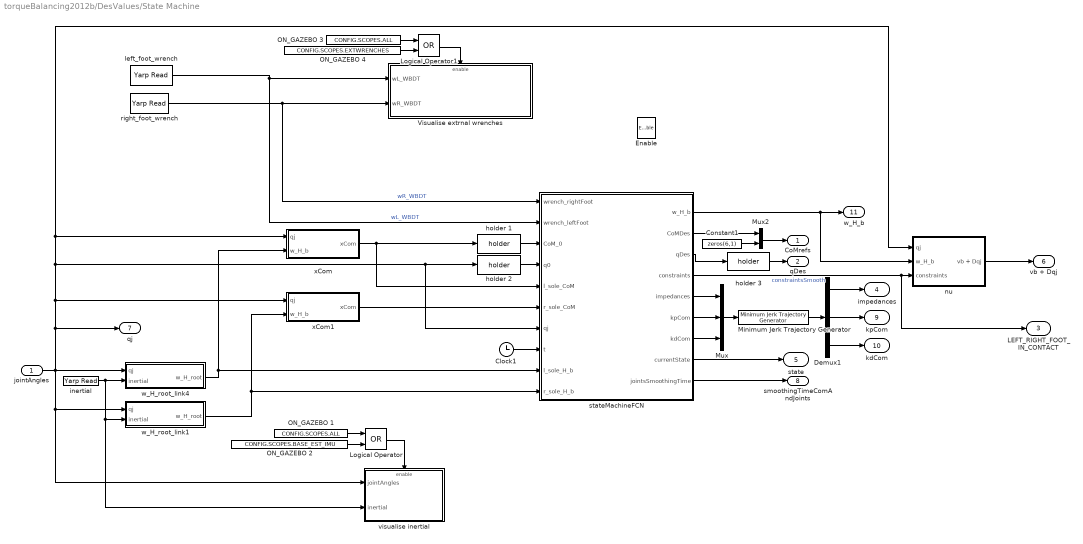
== system torqueBalancing2012b/DesValues/State Machine ==
  jointAngles : Inport
  Enable : EnablePort
  Clock1 : Clock
  Constant1 : Constant  Value=zeros(6,1)
  Demux1 : Demux  Outputs=[ROBOT_DOF,3,3]
  Logical Operator : Logic  Operator=OR  AllPortsSameDT=off  OutDataTypeStr=boolean
  Logical Operator1 : Logic  Operator=OR  AllPortsSameDT=off  OutDataTypeStr=boolean
  Minimum Jerk Trajectory Generator : WBToolboxLibrary/Utilities/Minimum Jerk Trajectory Generator  externalSettlingTime=off  settlingTime=gain.SmoothingTimeGainScheduling  sampleTime=CONFIG.Ts  firstDerivatives=off  secondDerivatives=off  explicitInitialValue=off
  Mux : Mux  Inputs=3
  Mux2 : Mux  Inputs=2
  ON_GAZEBO 1 : Constant  Value=CONFIG.SCOPES.ALL
  ON_GAZEBO 2 : Constant  Value=CONFIG.SCOPES.BASE_EST_IMU
  ON_GAZEBO 3 : Constant  Value=CONFIG.SCOPES.ALL
  ON_GAZEBO 4 : Constant  Value=CONFIG.SCOPES.EXTWRENCHES
  "Visualise extrnal wrenches  " : Subsystem
  holder 1 : WBToolboxLibrary/Utilities/holder 
  holder 2 : WBToolboxLibrary/Utilities/holder 
  holder 3 : WBToolboxLibrary/Utilities/holder 
  inertial : WBToolboxLibrary/Utilities/Yarp Read  portName=PORTS.IMU  signalSize=12  blocking=off  timestamp=off  autoconnect=on  errorOnConnection=on
  left_foot_wrench : WBToolboxLibrary/Utilities/Yarp Read  portName=PORTS.WBDT_LEFTLEG_EE  signalSize=6  blocking=off  timestamp=off  autoconnect=on  errorOnConnection=off
  nu : Subsystem
  right_foot_wrench : WBToolboxLibrary/Utilities/Yarp Read  portName=PORTS.WBDT_RIGHTLEG_EE  signalSize=6  blocking=off  timestamp=off  autoconnect=on  errorOnConnection=off
  stateMachineFCN : MATLAB Function  TreatAsAtomicUnit=on
      settings: PermitHierarchicalResolution=ParametersOnly
  visualise inertial : Subsystem
  w_H_root_link1 : Subsystem  mask{link_name='r_sole'}
      mask prompts: link_name "link name"
      mask help:
      | This block evaluates the homogeneous transformation between the world and the root link, i.e. ^wH_b. It assumes that the link specified by the variable 'link_name' has a constant position
      | w.r.t. an inertial frame, but it can rotate arbitrarily. This rotation is retrived from the IMU sensor.
      mask Display:
      | str = strrep(link_name, '_','\_');
      | port_label('output',1,['{}^{',str '}H_{root}'],'texmode','on')
      | clear str;
      | 
      | port_label('input',1,'q_j','texmode','on')
      | 
      | port_label('input',2,'inertial','texmode','on')
  w_H_root_link4 : Subsystem  mask{link_name='l_sole'}
      mask prompts: link_name "link name"
      mask help:
      | This block evaluates the homogeneous transformation between the world and the root link, i.e. ^wH_b. It assumes that the link specified by the variable 'link_name' has a constant position
      | w.r.t. an inertial frame, but it can rotate arbitrarily. This rotation is retrived from the IMU sensor.
      mask Display:
      | str = strrep(link_name, '_','\_');
      | port_label('output',1,['{}^{',str '}H_{root}'],'texmode','on')
      | clear str;
      | 
      | port_label('input',1,'q_j','texmode','on')
      | 
      | port_label('input',2,'inertial','texmode','on')
  xCom : Subsystem
  xCom1 : Subsystem
  CoMrefs : Outport
  qDes : Outport  Port=2
  LEFT_RIGHT_FOOT_IN_CONTACT : Outport  Port=3
  impedances : Outport  Port=4
  state : Outport  Port=5
  vb + Dqj : Outport  Port=6
  qj : Outport  Port=7
  smoothingTimeComAndJoints : Outport  Port=8
  kpCom : Outport  Port=9
  kdCom : Outport  Port=10
  w_H_b : Outport  Port=11
  wires:
  right_foot_wrench/1 -> "Visualise extrnal wrenches  "/2(wR_WBDT), stateMachineFCN/1(wrench_rightFoot)  "wR_WBDT"
  xCom/1(xCom) -> stateMachineFCN/5(l_sole_CoM), holder 1/1
  holder 1/1 -> stateMachineFCN/3(CoM_0)
  holder 2/1 -> stateMachineFCN/4(q0)
  Clock1/1 -> stateMachineFCN/8(t)
  stateMachineFCN/3(qDes) -> holder 3/1
  stateMachineFCN/2(CoMDes) -> Mux2/1
  Mux2/1 -> CoMrefs/1
  Constant1/1 -> Mux2/2
  stateMachineFCN/8(currentState) -> state/1
  stateMachineFCN/4(constraints) -> LEFT_RIGHT_FOOT_IN_CONTACT/1, nu/3("constraints ")  "constraintsSmooth"
  left_foot_wrench/1 -> "Visualise extrnal wrenches  "/1(wL_WBDT), stateMachineFCN/2(wrench_leftFoot)  "wL_WBDT"
  stateMachineFCN/1(w_H_b) -> w_H_b/1, nu/2(w_H_b)
  xCom1/1(xCom) -> stateMachineFCN/6(r_sole_CoM)
  nu/1(vb + Dqj) -> vb + Dqj/1
  w_H_root_link4/1(w_H_root) -> stateMachineFCN/9(l_sole_H_b), xCom/2(w_H_b)
  w_H_root_link1/1(w_H_root) -> stateMachineFCN/10(r_sole_H_b), xCom1/2(w_H_b)
  jointAngles/1 -> w_H_root_link4/1(qj), w_H_root_link1/1(qj), visualise inertial/1(jointAngles), nu/1(qj), xCom/1(qj), stateMachineFCN/7(qj), holder 2/1, xCom1/1(qj), qj/1
  inertial/1 -> w_H_root_link1/2(inertial), visualise inertial/2(inertial), w_H_root_link4/2(inertial)
  stateMachineFCN/9(jointsSmoothingTime) -> smoothingTimeComAndJoints/1
  Logical Operator1/1 -> "Visualise extrnal wrenches  "/Enable
  ON_GAZEBO 1/1 -> Logical Operator/1
  ON_GAZEBO 2/1 -> Logical Operator/2
  Logical Operator/1 -> visualise inertial/Enable
  ON_GAZEBO 3/1 -> Logical Operator1/1
  ON_GAZEBO 4/1 -> Logical Operator1/2
  stateMachineFCN/6(kpCom) -> Mux/2
  Demux1/3 -> kdCom/1
  stateMachineFCN/7(kdCom) -> Mux/3
  stateMachineFCN/5(impedances) -> Mux/1
  Mux/1 -> Minimum Jerk Trajectory Generator/1
  Minimum Jerk Trajectory Generator/1 -> Demux1/1
  Demux1/1 -> impedances/1
  Demux1/2 -> kpCom/1
  holder 3/1 -> qDes/1

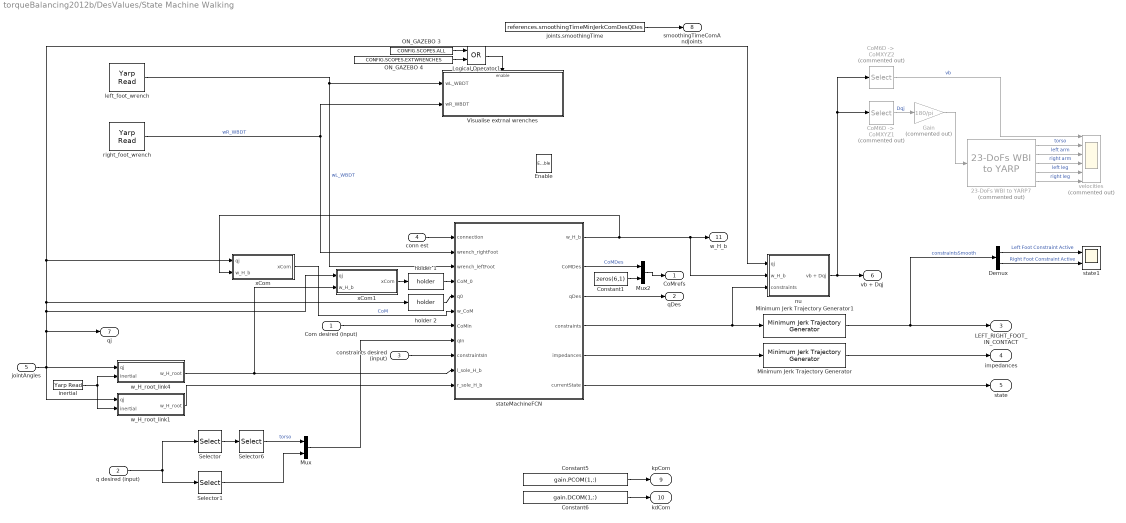
== system torqueBalancing2012b/DesValues/State Machine Walking ==
  Com desired (input) : Inport
  q desired (input) : Inport  Port=2
  constraints desired (input) : Inport  Port=3
  conn est : Inport  Port=4
  jointAngles : Inport  Port=5
  Enable : EnablePort
  23-DoFs WBI to YARP7 : WBToolboxLibrary/Utilities/23-DoFs WBI to YARP  Commented=on
  "CoM6D ->  CoMXYZ1" : Selector  Commented=on  InputPortWidth=ROBOT_DOF+6  IndexOptions=Index vector (dialog)  Indices=[7:ROBOT_DOF+6]  OutputSizes=1
  "CoM6D ->  CoMXYZ2" : Selector  Commented=on  InputPortWidth=ROBOT_DOF+6  IndexOptions=Index vector (dialog)  Indices=[1 2 3 4 5 6]  OutputSizes=1
  Constant1 : Constant  Value=zeros(6,1)
  Constant5 : Constant  Value=gain.PCOM(1,:)
  Constant6 : Constant  Value=gain.DCOM(1,:)
  Demux : Demux  Outputs=2
  Gain : Gain  Commented=on  Gain=180/pi
  Logical Operator1 : Logic  Operator=OR  AllPortsSameDT=off  OutDataTypeStr=boolean
  Minimum Jerk Trajectory Generator : WBToolboxLibrary/Utilities/Minimum Jerk Trajectory Generator  externalSettlingTime=off  settlingTime=gain.SmoothingTimeImp  sampleTime=CONFIG.Ts  firstDerivatives=off  secondDerivatives=off  explicitInitialValue=off
  Minimum Jerk Trajectory Generator1 : WBToolboxLibrary/Utilities/Minimum Jerk Trajectory Generator  externalSettlingTime=off  settlingTime=CONFIG.smoothingTimeTranDynamics  sampleTime=CONFIG.Ts  firstDerivatives=off  secondDerivatives=off  explicitInitialValue=off
  Mux : Mux  Inputs=2
  Mux2 : Mux  Inputs=2
  ON_GAZEBO 3 : Constant  Value=CONFIG.SCOPES.ALL
  ON_GAZEBO 4 : Constant  Value=CONFIG.SCOPES.EXTWRENCHES
  Selector : Selector  InputPortWidth=ROBOT_DOF  IndexOptions=Index vector (dialog)  Indices=[1:3]  OutputSizes=1
  Selector1 : Selector  InputPortWidth=ROBOT_DOF  IndexOptions=Index vector (dialog)  Indices=[4:ROBOT_DOF]  OutputSizes=1
  Selector6 : Selector  InputPortWidth=3  IndexOptions=Index vector (dialog)  Indices=[3 2 1]  OutputSizes=1
  "Visualise extrnal wrenches  " : Subsystem
  holder 1 : WBToolboxLibrary/Utilities/holder 
  holder 2 : WBToolboxLibrary/Utilities/holder 
  inertial : WBToolboxLibrary/Utilities/Yarp Read  portName=PORTS.IMU  signalSize=12  blocking=off  timestamp=off  autoconnect=on  errorOnConnection=off
  joints.smoothingTime : Constant  Value=references.smoothingTimeMinJerkComDesQDes
  left_foot_wrench : WBToolboxLibrary/Utilities/Yarp Read  portName=PORTS.WBDT_LEFTLEG_EE  signalSize=6  blocking=off  timestamp=off  autoconnect=on  errorOnConnection=off
  nu : Subsystem
  right_foot_wrench : WBToolboxLibrary/Utilities/Yarp Read  portName=PORTS.WBDT_RIGHTLEG_EE  signalSize=6  blocking=off  timestamp=off  autoconnect=on  errorOnConnection=off
  state1 : Scope  NumInputPorts=2
      settings: TimeRange=auto  LimitDataPoints=on  MaxDataPoints=5000  SaveToWorkspace=off  SaveName=ScopeData2  YMin=-0.14635~-0.14635  YMax=1.12737~1.12737  SampleTime=-1  DataFormat=Array
  stateMachineFCN : MATLAB Function  Priority=-1  TreatAsAtomicUnit=on
      settings: PermitHierarchicalResolution=ParametersOnly
  velocities : Scope  Commented=on  NumInputPorts=6
      settings: TimeRange=auto  MaxDataPoints=5000  SaveToWorkspace=off  SaveName=ScopeData2  YMin=-2.14738~-2.14738~-2.14738~-2.14738~-2.14738~-2.14738  YMax=2.60944~2.60944~2.60944~2.60944~2.60944~2.60944  SampleTime=-1
  w_H_root_link1 : Subsystem  mask{link_name='r_sole'}
      mask prompts: link_name "link name"
      mask help:
      | This block evaluates the homogeneous transformation between the world and the root link, i.e. ^wH_b. It assumes that the link specified by the variable 'link_name' has a constant position
      | w.r.t. an inertial frame, but it can rotate arbitrarily. This rotation is retrived from the IMU sensor.
      mask Display:
      | str = strrep(link_name, '_','\_');
      | port_label('output',1,['{}^{',str '}H_{root}'],'texmode','on')
      | clear str;
      | 
      | port_label('input',1,'q_j','texmode','on')
      | 
      | port_label('input',2,'inertial','texmode','on')
  w_H_root_link4 : Subsystem  mask{link_name='l_sole'}
      mask prompts: link_name "link name"
      mask help:
      | This block evaluates the homogeneous transformation between the world and the root link, i.e. ^wH_b. It assumes that the link specified by the variable 'link_name' has a constant position
      | w.r.t. an inertial frame, but it can rotate arbitrarily. This rotation is retrived from the IMU sensor.
      mask Display:
      | str = strrep(link_name, '_','\_');
      | port_label('output',1,['{}^{',str '}H_{root}'],'texmode','on')
      | clear str;
      | 
      | port_label('input',1,'q_j','texmode','on')
      | 
      | port_label('input',2,'inertial','texmode','on')
  xCom : Subsystem  Priority=-2
  xCom1 : Subsystem  Priority=-2
  CoMrefs : Outport
  qDes : Outport  Port=2
  LEFT_RIGHT_FOOT_IN_CONTACT : Outport  Port=3
  impedances : Outport  Port=4
  state : Outport  Port=5
  vb + Dqj : Outport  Port=6
  qj : Outport  Port=7
  smoothingTimeComAndJoints : Outport  Port=8
  kpCom : Outport  Port=9
  kdCom : Outport  Port=10
  w_H_b : Outport  Port=11
  wires:
  xCom/1(xCom) -> stateMachineFCN/6(w_CoM)  "CoM"
  holder 2/1 -> stateMachineFCN/5(q0)
  stateMachineFCN/3(qDes) -> qDes/1
  stateMachineFCN/2(CoMDes) -> Mux2/1  "CoMDes"
  Mux2/1 -> CoMrefs/1
  Constant1/1 -> Mux2/2
  stateMachineFCN/5(impedances) -> Minimum Jerk Trajectory Generator/1
  stateMachineFCN/6(currentState) -> state/1
  Minimum Jerk Trajectory Generator1/1 -> Demux/1, LEFT_RIGHT_FOOT_IN_CONTACT/1  "constraintsSmooth"
  stateMachineFCN/4(constraints) -> nu/3("constraints "), Minimum Jerk Trajectory Generator1/1
  Demux/1 -> state1/1  "Left Foot Constraint Active"
  Demux/2 -> state1/2  "Right Foot Constraint Active"
  stateMachineFCN/1(w_H_b) -> xCom/2(w_H_b), nu/2(w_H_b), w_H_b/1
  nu/1(vb + Dqj) -> vb + Dqj/1, "CoM6D ->  CoMXYZ1"/1, "CoM6D ->  CoMXYZ2"/1
  Minimum Jerk Trajectory Generator/1 -> impedances/1
  "CoM6D ->  CoMXYZ2"/1 -> velocities/1  "vb"
  "CoM6D ->  CoMXYZ1"/1 -> Gain/1  "Dqj"
  23-DoFs WBI to YARP7/1 -> velocities/2  "torso"
  23-DoFs WBI to YARP7/2 -> velocities/3  "left arm"
  23-DoFs WBI to YARP7/3 -> velocities/4  "right arm"
  23-DoFs WBI to YARP7/4 -> velocities/5  "left leg"
  23-DoFs WBI to YARP7/5 -> velocities/6  "right leg"
  Gain/1 -> 23-DoFs WBI to YARP7/1
  w_H_root_link4/1(w_H_root) -> stateMachineFCN/10(l_sole_H_b), xCom1/2(w_H_b)
  w_H_root_link1/1(w_H_root) -> stateMachineFCN/11(r_sole_H_b)
  jointAngles/1 -> w_H_root_link1/1(qj), w_H_root_link4/1(qj), nu/1(qj), xCom/1(qj), holder 2/1, xCom1/1(qj), qj/1
  inertial/1 -> w_H_root_link1/2(inertial), w_H_root_link4/2(inertial)
  Com desired (input)/1 -> stateMachineFCN/7(CoMIn)
  constraints desired (input)/1 -> stateMachineFCN/9(constraintsIn)
  holder 1/1 -> stateMachineFCN/4(CoM_0)
  xCom1/1(xCom) -> holder 1/1
  conn est/1 -> stateMachineFCN/1(connection)
  q desired (input)/1 -> Selector/1, Selector1/1
  Selector6/1 -> Mux/1  "torso"
  Selector/1 -> Selector6/1
  Selector1/1 -> Mux/2
  Mux/1 -> stateMachineFCN/8(qIn)
  joints.smoothingTime/1 -> smoothingTimeComAndJoints/1
  right_foot_wrench/1 -> stateMachineFCN/2(wrench_rightFoot), "Visualise extrnal wrenches  "/2(wR_WBDT)  "wR_WBDT"
  left_foot_wrench/1 -> "Visualise extrnal wrenches  "/1(wL_WBDT), stateMachineFCN/3(wrench_leftFoot)  "wL_WBDT"
  Logical Operator1/1 -> "Visualise extrnal wrenches  "/Enable
  ON_GAZEBO 3/1 -> Logical Operator1/1
  ON_GAZEBO 4/1 -> Logical Operator1/2
  Constant5/1 -> kpCom/1
  Constant6/1 -> kdCom/1

== system torqueBalancing2012b/DesValues/Subsystem ==
  conn status 1 : Inport
  conn status 2 : Inport  Port=2
  conn status 3 : Inport  Port=3
  Compare To Zero3 : simulink/Logic and Bit Operations/Compare To Zero  relop=>  OutDataTypeStr=boolean
  Compare To Zero4 : simulink/Logic and Bit Operations/Compare To Zero  relop=>  OutDataTypeStr=boolean
  Compare To Zero5 : simulink/Logic and Bit Operations/Compare To Zero  relop=>  OutDataTypeStr=boolean
  Logical Operator : Logic  Inputs=3  AllPortsSameDT=off  OutDataTypeStr=boolean
  connection check : Outport
  wires:
  Logical Operator/1 -> connection check/1
  Compare To Zero4/1 -> Logical Operator/3
  conn status 1/1 -> Compare To Zero3/1
  Compare To Zero3/1 -> Logical Operator/1
  conn status 3/1 -> Compare To Zero4/1
  Compare To Zero5/1 -> Logical Operator/2
  conn status 2/1 -> Compare To Zero5/1

== system torqueBalancing2012b/Dump and visualize/ZMPs ==
  fDesQP : Inport
  Demux1 : Demux  Outputs=3
  Demux2 : Demux  Outputs=3
  Divide{4..7} (4 alike) : Product  Inputs=*/
  Gain3 : Gain  Gain=-1
  Gain4 : Gain  Gain=-1
  Mux : Mux  Inputs=2
  Mux1 : Mux  Inputs=2
  fz taux tauy Left : Selector  InputPortWidth=12  IndexOptions=Index vector (dialog)  Indices=[3 4 5]  OutputSizes=1
  fz taux tauy Right : Selector  InputPortWidth=12  IndexOptions=Index vector (dialog)  Indices=[9 10 11]  OutputSizes=1
  ZMP_LeftFoot : Outport
  ZMP_RightFoot : Outport  Port=2
  wires:
  fz taux tauy Left/1 -> Demux1/1
  Demux1/1 -> Divide4/2, Divide5/2
  Divide7/1 -> Gain4/1
  Divide4/1 -> Mux/2
  Divide5/1 -> Gain3/1
  fz taux tauy Right/1 -> Demux2/1
  Demux2/1 -> Divide6/2, Divide7/2
  fDesQP/1 -> fz taux tauy Left/1, fz taux tauy Right/1
  Gain3/1 -> Mux/1
  Mux/1 -> ZMP_LeftFoot/1
  Divide6/1 -> Mux1/2
  Gain4/1 -> Mux1/1
  Mux1/1 -> ZMP_RightFoot/1
  Demux1/2 -> Divide4/1  "tauxL"
  Demux1/3 -> Divide5/1  "tauyL"
  Demux2/2 -> Divide6/1  "tauxR"
  Demux2/3 -> Divide7/1  "tauyR"

== system torqueBalancing2012b/Dump and visualize/plotNorms ==
  qTile_LeftLeg : Inport
  qTile_RightLeg : Inport  Port=2
  state : Inport  Port=3
  Constant : Constant  Value=sm.joints.thresholdInContact
  Constant2 : Constant  Value=sm.joints.thresholdNotInContact
  Mux : Mux  Inputs=3
  Mux1 : Mux  Inputs=3
  norm : MATLAB Function  TreatAsAtomicUnit=on
      settings: PermitHierarchicalResolution=ParametersOnly
  norm(qTilde) : Scope  NumInputPorts=3
      settings: TimeRange=auto  ShowLegends=on  MaxDataPoints=5000  SaveToWorkspace=off  YMin=-6.25~-6.25~-6.25  YMax=56.25~56.25~56.25  SampleTime=-1
  norm1 : MATLAB Function  TreatAsAtomicUnit=on
      settings: PermitHierarchicalResolution=ParametersOnly
  wires:
  Constant/1 -> Mux1/2, Mux/2  "thresholdInContact"
  qTile_LeftLeg/1 -> norm1/1(u)
  qTile_RightLeg/1 -> norm/1(u)
  norm/1(normU) -> Mux1/1  "norm(qTilde_RightL)"
  norm1/1(normU) -> Mux/1  "norm(qTilde_LeftL)"
  Mux/1 -> norm(qTilde)/1
  Mux1/1 -> norm(qTilde)/2
  Constant2/1 -> Mux1/3, Mux/3  "thresholdNotInContact"
  state/1 -> norm(qTilde)/3
